simulink library "vehdynlibeom_TUM"  (R2018b)
settings: Solver=VariableStepAuto  StartTime=0.0  StopTime=10.0  RelTol=1e-3
libraries: autolibsharedcommon x7, shared6dof x4, shared6dofsys x3, autolibshared x2, sharedutil x2, sharedtransform x1
Description:
  | Vehicle Dynamics Blockset: Equations of Motion
  | Copyright 2017 The MathWorks Inc.
settings Model: ModifiedByFormat=The MathWorks, Inc.  Creator=The MathWorks, Inc.  LastModifiedBy=The MathWorks, Inc.
settings DebuggingCC: LibraryContextMissingDiagnostic=none
settings SFSimCC: SimUseLocalCustomCode=off
settings RTWCC: RTWUseLocalCustomCode=off
settings CodeAppCC: StateflowObjectComments=on

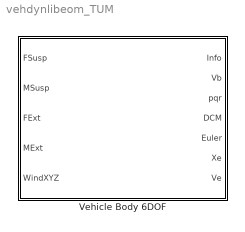
== system vehdynlibeom_TUM ==
  Vehicle Body 6DOF : Subsystem  mask(Vehicle Body 6DOF 2 Axle){m=2000, a=1.4, b=1.6, d=0, h=0.35, Xe0=0, Ye0=0, Ze0=0, vx0_mps=0, vy0_mps=0, vz0_mps=0, phi0_rad=0, theta0_rad=0, psi0_rad=0, phidot0_radps=0, thetadot0_radps=0, psidot0_radps=0, Iveh=[430 0 0; 0 1900 0; 0 0 2100], tw_front=1.8, tw_rear=1.9, z1m=0, z1R=[-.25,.125,.15], z1I=[1.4,-.2,.1;-.2,1.4,.1;.1,.1,2.25].*0, z2m=0, z2R=[1.4,0,.8], z2I=[1.4,-.2,.1;-.2,1.4,.1;.1,.1,2.25].*0, z3m=0, z3R=[.75,-.5,.4], z3I=[5,-.1,-2;-2,9,.1;-.1,.1,6].*0, z4m=0, z4R=[.75,.5,.4], z4I=[5,-.1,-2;-2,9,.1;-.1,.1,6].*0, z5m=0, z5R=[1.25,-.5,.4], z5I=[5,-.1,-2;-2,9,.1;-.1,.1,6].*0, z6m=0, z6R=[1.25,-.5,.4], z6I=[5,-.1,-2;-2,9,.1;-.1,.1,6].*0, z7m=0, z7R=[2,0,.25], z7I=[1.4,-.2,.1;-.2,1.4,.1;.1,.1,2.25].*0, Af=2, Cd=.3, Cl=.1, Cpm=.1, beta_w=[0:0.001:0.01], Cs=[0:0.01:0.1], Cym=[0:0.001:0.01], sign_cl=0, Pabs=101325, Tair=273, g=9.81, xdot_tol=.1, longOff=0, latOff=0, vertOff=0, aMode=2}
      mask prompts: m "vdynblks:vehdynVehBody6Dof:blkPrm_m"; a "vdynblks:vehdynVehBody6Dof:blkPrm_a"; b "vdynblks:vehdynVehBody6Dof:blkPrm_b"; d "vdynblks:vehdynVehBody6Dof:blkPrm_d"; h "vdynblks:vehdynVehBody6Dof:blkPrm_h"; Xe0 "Initial position in intertial frame Xe0_m [m]"; Ye0 "Initial position in intertial frame Ye0_m [m]"; Ze0 "Initial position in intertial frame Ze0_m [m]"; vx0_mps "Initial velocity vx0_mps [m/s]"; vy0_mps "Initial velocity vy0_mps [m/s]"; vz0_mps "Initial velocity vz0_mps [m/s]"; phi0_rad "Initial Euler angle roll, phi0_rad [rad]"; theta0_rad "Initial Euler angle pitch, theta0_rad [rad]"; psi0_rad "Initial Euler angle yaw, psi0_rad [rad]"; phidot0_radps "Initial body rotation rates phidot0_radps [rad/s]"; thetadot0_radps "Initial body rotation rates theta0_radps [rad/s]"; psidot0_radps "Initial body rotation rates psidot0_radps [rad/s]"; Iveh "vdynblks:vehdynVehBody6Dof:blkPrm_Iveh"; tw_front "Track width front, tw_front [m];"; tw_rear "Track width rear, tw_rear [m];"; z1m "vdynblks:vehdynVehBody6Dof:blkPrm_z1m"; z1R "vdynblks:vehdynVehBody6Dof:blkPrm_z1R"; z1I "vdynblks:vehdynVehBody6Dof:blkPrm_z1I"; z2m "vdynblks:vehdynVehBody6Dof:blkPrm_z2m"; z2R "vdynblks:vehdynVehBody6Dof:blkPrm_z2R"; z2I "vdynblks:vehdynVehBody6Dof:blkPrm_z2I"; z3m "vdynblks:vehdynVehBody6Dof:blkPrm_z3m"; z3R "vdynblks:vehdynVehBody6Dof:blkPrm_z3R"; z3I "vdynblks:vehdynVehBody6Dof:blkPrm_z3I"; z4m "vdynblks:vehdynVehBody6Dof:blkPrm_z4m"; z4R "vdynblks:vehdynVehBody6Dof:blkPrm_z4R"; z4I "vdynblks:vehdynVehBody6Dof:blkPrm_z4I"; z5m "vdynblks:vehdynVehBody6Dof:blkPrm_z5m"; z5R "vdynblks:vehdynVehBody6Dof:blkPrm_z5R"; z5I "vdynblks:vehdynVehBody6Dof:blkPrm_z5I"; z6m "vdynblks:vehdynVehBody6Dof:blkPrm_z6m"; z6R "vdynblks:vehdynVehBody6Dof:blkPrm_z6R"; z6I "vdynblks:vehdynVehBody6Dof:blkPrm_z6I"; z7m "vdynblks:vehdynVehBody6Dof:blkPrm_z7m"; z7R "vdynblks:vehdynVehBody6Dof:blkPrm_z7R"; z7I "vdynblks:vehdynVehBody6Dof:blkPrm_z7I"; Af "vdynblks:vehdynVehBody6Dof:blkPrm_Af"; Cd "vdynblks:vehdynVehBody6Dof:blkPrm_Cd"; Cl "vdynblks:vehdynVehBody6Dof:blkPrm_Cl"; Cpm "vdynblks:vehdynVehBody6Dof:blkPrm_Cpm"; beta_w "vdynblks:vehdynVehBody6Dof:blkPrm_beta_w"; Cs "vdynblks:vehdynVehBody6Dof:blkPrm_Cs"; Cym "vdynblks:vehdynVehBody6Dof:blkPrm_Cym"; sign_cl "Long. lift coeff. sign, sign_cl [-]:"; Pabs "vdynblks:vehdynVehBody6Dof:blkPrm_Pabs"; Tair "vdynblks:vehdynVehBody6Dof:blkPrm_Tair"; g "vdynblks:vehdynVehBody6Dof:blkPrm_g"; xdot_tol "vdynblks:vehdynVehBody6Dof:blkPrm_xdot_tol"; longOff "vdynblks:vehdynVehBody6Dof:blkPrm_longOff"; latOff "vdynblks:vehdynVehBody6Dof:blkPrm_latOff"; vertOff "vdynblks:vehdynVehBody6Dof:blkPrm_vertOff"
      mask help: vdynblks:vehdynVehBody6Dof:blkDesc
      mask init:
      | dummy = 1;
      mask Help: eval('vdynblkshelp(''vb6dof'')')
      mask DialogControl vehLayoutPanel Prompt: vdynblks:vehdynVehBody6Dof:blkDlg_Container28
      mask DialogControl LongPanel Prompt: vdynblks:vehdynVehBody6Dof:blkDlg_LongPanel
      mask DialogControl m Prompt: Vehicle mass, m [kg]:
      mask DialogControl a Prompt: Longitudinal distance from center of mass to front axle, a [m]:
      mask DialogControl b Prompt: Longitudinal distance from center of mass to rear axle, b [m]:
      mask DialogControl d Prompt: Lateral distance from geometric centerline to center of mass, d [m]:
      mask DialogControl h Prompt: Vertical distance from center of mass to axle plane, h [m]:
      mask DialogControl Iveh Prompt: Chassis inertia tensor, Iveh [kg*m^2]:
      mask DialogControl loadPanel Prompt: vdynblks:vehdynVehBody6Dof:blkDlg_loadPanel
      mask DialogControl zone1Panel Prompt: vdynblks:vehdynVehBody6Dof:blkDlg_zone1Panel
      mask DialogControl z1m Prompt: Mass, z1m [kg]:
      mask DialogControl z1R Prompt: Distance vector from front axle, z1R [m]:
      mask DialogControl z1I Prompt: Inertia tensor, z1I, [kg*m^2]:
      mask DialogControl zone2Panel Prompt: vdynblks:vehdynVehBody6Dof:blkDlg_zone2Panel
      mask DialogControl z2m Prompt: Mass, z2m [kg]:
      mask DialogControl z2R Prompt: Distance vector from front axle, z2R [m]:
      mask DialogControl z2I Prompt: Inertia tensor, z2I, [kg*m^2]:
      mask DialogControl zone3Panel Prompt: vdynblks:vehdynVehBody6Dof:blkDlg_zone3Panel
      mask DialogControl z3m Prompt: Mass, z3m [kg]:
      mask DialogControl z3R Prompt: Distance vector from front axle, z3R [m]:
      mask DialogControl z3I Prompt: Inertia tensor, z3I, [kg*m^2]:
      mask DialogControl zone4Panel Prompt: vdynblks:vehdynVehBody6Dof:blkDlg_zone4Panel
      mask DialogControl z4m Prompt: Mass, z4m [kg]:
      mask DialogControl z4R Prompt: Distance vector from front axle, z4R [m]:
      mask DialogControl z4I Prompt: Inertia tensor, z4I, [kg*m^2]:
      mask DialogControl zone5Panel Prompt: vdynblks:vehdynVehBody6Dof:blkDlg_zone5Panel
      mask DialogControl z5m Prompt: Mass, z5m [kg]:
      mask DialogControl z5R Prompt: Distance vector from front axle, z5R [m]:
      mask DialogControl z5I Prompt: Inertia tensor, z5I, [kg*m^2]:
      mask DialogControl zone6Panel Prompt: vdynblks:vehdynVehBody6Dof:blkDlg_zone6Panel
      mask DialogControl z6m Prompt: Mass, z6m [kg]:
      mask DialogControl z6R Prompt: Distance vector from front axle, z6R [m]:
      mask DialogControl z6I Prompt: Inertia tensor, z6I, [kg*m^2]:
      mask DialogControl zone7Panel Prompt: vdynblks:vehdynVehBody6Dof:blkDlg_zone7Panel
      mask DialogControl z7m Prompt: Mass, z7m [kg]:
      mask DialogControl z7R Prompt: Distance vector from front axle, z7R [m]:
      mask DialogControl z7I Prompt: Inertia tensor, z7I, [kg*m^2]:
      mask DialogControl AeroParams Prompt: vdynblks:vehdynVehBody6Dof:blkDlg_AeroParams
      mask DialogControl Af Prompt: Longitudinal drag area, Af [m^2]:
      mask DialogControl Cd Prompt: Longitudinal drag coefficient, Cd [-]:
      mask DialogControl Cl Prompt: Longitudinal lift coefficient, Cl [-]:
      mask DialogControl Cpm Prompt: Longitudinal drag pitch moment, Cpm [-]:
      mask DialogControl beta_w Prompt: Relative wind angle vector, beta_w [rad]:
      mask DialogControl Cs Prompt: Side force coefficient vector, Cs [-]:
      mask DialogControl Cym Prompt: Yaw moment coefficient vector, Cym [-]:
      mask DialogControl EnviroPanel Prompt: vdynblks:vehdynVehBody6Dof:blkDlg_EnviroPanel
      mask DialogControl Pabs Prompt: Absolute Pressure, Pabs [Pa]:
      mask DialogControl Tair Prompt: Air temperature, Tair [K]:
      mask DialogControl g Prompt: Gravitational acceleration, g [m/s^2]:
      mask DialogControl SimPanel Prompt: vdynblks:vehdynVehBody6Dof:blkDlg_SimPanel
      mask DialogControl xdot_tol Prompt: Longitudinal velocity tolerance, xdot_tol [m/s]:
      mask DialogControl longOff Prompt: Geometric longitudinal offset from axle plane, longOff [m]:
      mask DialogControl latOff Prompt: Geometric lateral offset from axle plane, latOff [m]:
      mask DialogControl vertOff Prompt: Geometric vertical offset from axle plane, vertOff [m]:
      mask Display:
      | try
      |     IconInfo = vehdynicon('vehdynlib6dofcar',gcb,8);
      | 
      |     image(IconInfo.image, IconInfo.position);
      | 
      |     for i = 1:numel(IconInfo.lconn)
      |         port_label('lconn', i, IconInfo.lconn{i})
      |     end
      | 
      |     for j = 1:numel(IconInfo.rconn)
      |         port_label('rconn', j, IconInfo.rconn{j})
      |     end
      | 
      |     for k = 1:numel(IconInfo.input)
      |         port_label('input', k, IconInfo.input{k})
      |     end
      | 
      |     for m = 1:numel(IconInfo.output)
      |         port_label('output', m, IconInfo.output{m})
      |     end
      | catch
      |     fprintf('Vehicle Body \n 6DOF Car')
      | end

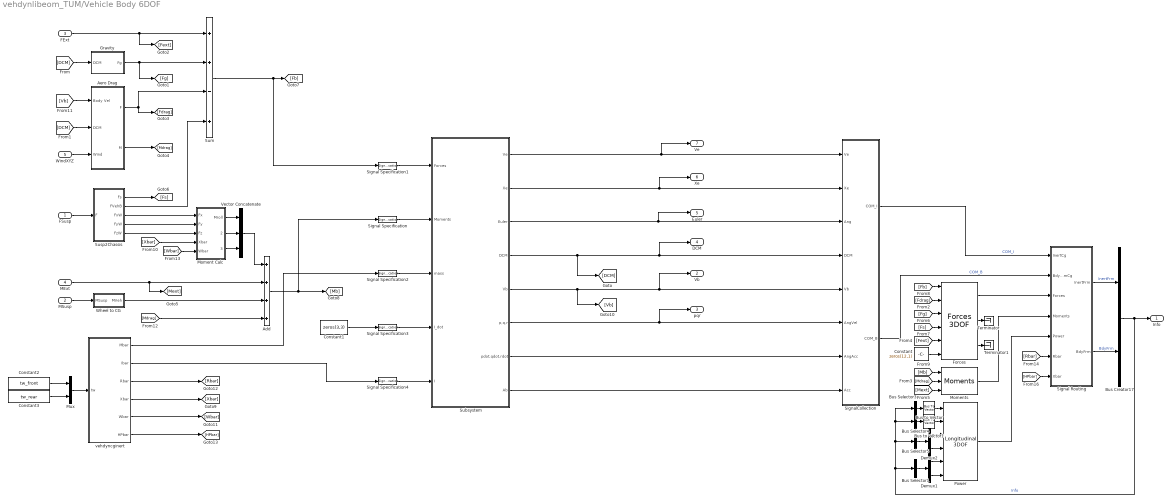
== system vehdynlibeom_TUM/Vehicle Body 6DOF ==
  FSusp : Inport  Unit=N
  MSusp : Inport  Port=2  Unit=N*m
  FExt : Inport  Port=3  Unit=N
  MExt : Inport  Port=4  Unit=N*m
  WindXYZ : Inport  Port=5  Unit=m/s
  Add : Sum  Inputs=++++
  Aero Drag : Subsystem
  Bus Creator17 : BusCreator  Inputs=2
  Bus Selector1 : BusSelector  OutputSignals=BdyFrm.Moments.Body.Mx,BdyFrm.Moments.Body.My,BdyFrm.Moments.Body.Mz,BdyFrm.Cg.AngVel.p,BdyFrm.Cg.AngVel.q,BdyFrm.Cg.AngVel.r  OutputAsBus=on
  Bus Selector3 : BusSelector  OutputSignals=BdyFrm.Forces.Body.Fx,BdyFrm.Forces.Body.Fy,BdyFrm.Forces.Body.Fz  OutputAsBus=on
  Bus Selector4 : BusSelector  OutputSignals=BdyFrm.Forces.Drag.Fx,BdyFrm.Forces.Drag.Fy,BdyFrm.Forces.Drag.Fz  OutputAsBus=on
  Bus Selector5 : BusSelector  OutputSignals=BdyFrm.Cg.Vel.xdot,BdyFrm.Cg.Vel.ydot,BdyFrm.Cg.Vel.zdot,BdyFrm.Moments.Drag.Mx,BdyFrm.Moments.Drag.My,BdyFrm.Moments.Drag.Mz  OutputAsBus=on
  Bus to Vector : BusToVector
  Bus to Vector1 : BusToVector
  Constant : Constant  Value=zeros(12,1)
  Constant1 : Constant  Value=zeros(3,3)
  Constant2 : Constant  Value=tw_front
  Constant3 : Constant  Value=tw_rear
  Demux1 : Demux  Outputs=[3, 3]
  Demux2 : Demux  Outputs=[3, 3]
  Forces : autolibshared/Vehicle Body 3DOF Single Track/Signal Routing/Signal Routing Dual/Forces 3DOF  SystemSampleTime=-1  VariantControl=2
      settings: SourceProductName=Powertrain Blockset  SourceProductBaseCode=PW
  Gravity : Subsystem
  Moment Calc : Subsystem
  Moments : autolibsharedcommon/Bus Creation/Moments  SystemSampleTime=-1
      settings: SourceProductName=Powertrain Blockset  SourceProductBaseCode=PW
  Mux : Mux  Inputs=2
  Power : autolibsharedcommon/Bus Creation/Power/Longitudinal 3DOF  SystemSampleTime=-1  VariantControl=2
      settings: SourceProductName=Powertrain Blockset  SourceProductBaseCode=PW
  Signal Routing : Subsystem  VariantControl=2
  Signal Specification : SignalSpecification  Dimensions=[3,1]
  Signal Specification1 : SignalSpecification  Dimensions=[3,1]
  Signal Specification2 : SignalSpecification  Dimensions=[1,1]
  Signal Specification3 : SignalSpecification  Dimensions=[3,3]
  Signal Specification4 : SignalSpecification  Dimensions=[3,3]
  SignalCollection : Subsystem
  Subsystem : Subsystem
  Sum : Sum  Inputs=++-+  SaturateOnIntegerOverflow=on  InputSameDT=on  OutDataTypeStr=Inherit: Same as first input
  Susp2Chassis : Subsystem
  Terminator : Terminator
  Terminator1 : Terminator
  Vector Concatenate : Concatenate  NumInputs=3
  Wheel to CG : Subsystem
  vehdyncginert : MATLAB Function  TreatAsAtomicUnit=on
  Info : Outport
  Vb : Outport  Port=2  Unit=m/s
  pqr : Outport  Port=3  Unit=rad/s
  DCM : Outport  Port=4
  Euler : Outport  Port=5  Unit=rad
  Xe : Outport  Port=6  Unit=m
  Ve : Outport  Port=7  Unit=m/s
  wires:
  Vector Concatenate/1 -> Add/1
  Susp2Chassis/1(Fs) -> [Fs]
  Moment Calc/3(Myaw) -> Vector Concatenate/3
  Moment Calc/1(Mroll) -> Vector Concatenate/1
  Moment Calc/2(Mpitch) -> Vector Concatenate/2
  MSusp/1 -> Wheel to CG/1(MSusp)
  FSusp/1 -> Susp2Chassis/1(F)
  Gravity/1(Fg) -> Sum/2, [Fg]
  Subsystem/7(pdot,qdot,rdot) -> SignalCollection/7(AngAcc)
  [DCM] -> Gravity/1(DCM)
  WindXYZ/1 -> Aero Drag/3(Wind)
  [Vb] -> Aero Drag/1(Body Vel)
  Add/1 -> [Mb], Signal Specification/1
  Subsystem/4(DCM) -> DCM/1, SignalCollection/4(DCM), [DCM]
  Aero Drag/2(M) -> [Mdrag]
  Aero Drag/1(F) -> [Fdrag], Sum/3
  [DCM] -> Aero Drag/2(DCM)
  Sum/1 -> Signal Specification1/1, [Fb]
  Subsystem/8(Ab) -> SignalCollection/8(Acc)
  FExt/1 -> [Fext], Sum/1
  Bus Selector1/1 -> Demux1/1
  Bus Selector3/1 -> Bus to Vector/1
  Demux2/2 -> Power/4
  Bus to Vector/1 -> Power/1
  Bus Selector5/1 -> Demux2/1
  Bus to Vector1/1 -> Power/2
  Demux2/1 -> Power/3
  Bus Selector4/1 -> Bus to Vector1/1
  Bus Creator17/1 -> Bus Selector3/1, Bus Selector4/1, Bus Selector5/1, Bus Selector1/1, Info/1  "Info"
  Demux1/2 -> Power/6
  Signal Routing/1(InertFrm) -> Bus Creator17/1  "InertFrm"
  Demux1/1 -> Power/5
  Power/1 -> Signal Routing/5(Power)
  Signal Routing/2(BdyFrm) -> Bus Creator17/2  "BdyFrm"
  SignalCollection/1(COM_I) -> Signal Routing/1(InertCg)  "COM_I"
  SignalCollection/2(COM_B) -> Signal Routing/2(BdyFrmCg)  "COM_B"
  Forces/1 -> Signal Routing/3(Forces)
  Moments/1 -> Signal Routing/4(Moments)
  [Fdrag] -> Forces/2
  [Mdrag] -> Moments/2
  [Fext] -> Forces/5
  [Mext] -> Moments/3
  [Fg] -> Forces/3
  [Fb] -> Forces/1
  [Mb] -> Moments/1
  Constant/1 -> Forces/6
  Forces/2 -> Terminator/1
  Forces/3 -> Terminator1/1
  Susp2Chassis/2(FVehB) -> Sum/4
  MExt/1 -> [Mext], Add/2
  Wheel to CG/1(MVeh) -> Add/3
  [Fs] -> Forces/4
  Susp2Chassis/3(FxW) -> Moment Calc/1(Fx)
  Susp2Chassis/4(FyW) -> Moment Calc/2(Fy)
  Susp2Chassis/5(FzW) -> Moment Calc/3(Fz)
  Subsystem/3(Euler) -> Euler/1, SignalCollection/3(Ang)
  Subsystem/5(Vb) -> SignalCollection/5(Vb), Vb/1, [Vb]
  Subsystem/6(p,q,r) -> SignalCollection/6(AngVel), pqr/1
  Subsystem/1(Ve) -> Ve/1, SignalCollection/1(Ve)
  Subsystem/2(Xe) -> Xe/1, SignalCollection/2(Xe)
  [Mdrag] -> Add/4
  vehdyncginert/1(Mbar) -> Signal Specification2/1
  vehdyncginert/3(Rbar) -> [Rbar]
  Constant1/1 -> Signal Specification3/1
  vehdyncginert/2(Ibar) -> Signal Specification4/1
  [Xbar] -> Moment Calc/4(Xbar)
  vehdyncginert/4(Xbar) -> [Xbar]
  vehdyncginert/5(Wbar) -> [Wbar]
  [Wbar] -> Moment Calc/5(Wbar)
  [HPbar] -> Signal Routing/7(Xbar)
  vehdyncginert/6(HPbar) -> [HPbar]
  [Rbar] -> Signal Routing/6(Rbar)
  Constant2/1 -> Mux/1
  Constant3/1 -> Mux/2
  Mux/1 -> vehdyncginert/1(tw)
  Signal Specification/1 -> Subsystem/2(Moments)
  Signal Specification1/1 -> Subsystem/1(Forces)
  Signal Specification2/1 -> Subsystem/3(mass)
  Signal Specification3/1 -> Subsystem/4(I_dot)
  Signal Specification4/1 -> Subsystem/5(I)

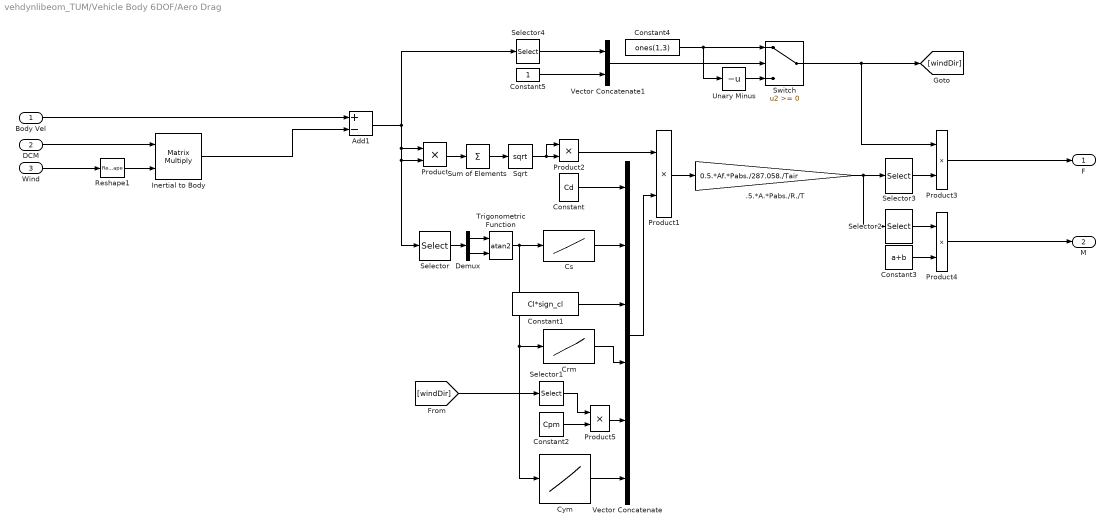
== system vehdynlibeom_TUM/Vehicle Body 6DOF/Aero Drag ==
  Body Vel : Inport
  DCM : Inport  Port=2
  Wind : Inport  Port=3
  .5.*A.*Pabs./R./T : Gain  Gain=0.5.*Af.*Pabs./287.058./Tair
  Add1 : Sum  Inputs=+-
  Constant : Constant  Value=Cd
  Constant1 : Constant  Value=Cl*sign_cl
  Constant2 : Constant  Value=Cpm
  Constant3 : Constant  Value=a+b
  Constant4 : Constant  Value=ones(1,3)
  Constant5 : Constant
  Crm : Lookup_n-D  NumberOfTableDimensions=1  BreakpointsForDimension1=[-1 1]  Table=[0 0]  InternalRulePriority=Speed  RndMeth=Simplest  InputSameDT=on
  Cs : Lookup_n-D  NumberOfTableDimensions=1  BreakpointsForDimension1=beta_w  Table=Cs  ExtrapMethod=Clip  InternalRulePriority=Speed  RndMeth=Simplest  InputSameDT=on
  Cym : Lookup_n-D  NumberOfTableDimensions=1  BreakpointsForDimension1=beta_w  Table=Cym  InternalRulePriority=Speed  RndMeth=Simplest  InputSameDT=on
  Demux : Demux  Outputs=2
  Inertial to Body : Product  Multiplication=Matrix(*)  SaturateOnIntegerOverflow=on  InputSameDT=on  OutDataTypeStr=Inherit: Same as first input
  Product{,1..5} (6 alike) : Product
  Reshape1 : Reshape
  Selector : Selector  InputPortWidth=3  IndexOptions=Index vector (dialog)  Indices=[2 1]  OutputSizes=1
  Selector1 : Selector  InputPortWidth=3  IndexOptions=Index vector (dialog)  Indices=[1]  OutputSizes=1
  Selector2 : Selector  InputPortWidth=6  IndexOptions=Index vector (dialog)  Indices=[4:6]  OutputSizes=1
  Selector3 : Selector  InputPortWidth=6  IndexOptions=Index vector (dialog)  Indices=[1:3]  OutputSizes=1
  Selector4 : Selector  InputPortWidth=3  IndexOptions=Index vector (dialog)  Indices=[1:2]  OutputSizes=1
  Sqrt : Sqrt  SaturateOnIntegerOverflow=on
  Sum of Elements : Sum  Inputs=+
  Switch : Switch  ZeroCross=off
  Trigonometric Function : Trigonometry  Operator=atan2  OutputSignalType=real
  Unary Minus : UnaryMinus
  Vector Concatenate : Concatenate  NumInputs=6
  Vector Concatenate1 : Concatenate
  F : Outport
  M : Outport  Port=2
  wires:
  Reshape1/1 -> Inertial to Body/2
  DCM/1 -> Inertial to Body/1
  Wind/1 -> Reshape1/1
  Constant4/1 -> Switch/1, Unary Minus/1
  Vector Concatenate1/1 -> Switch/2
  Crm/1 -> Vector Concatenate/4
  Constant5/1 -> Vector Concatenate1/2
  Selector3/1 -> Product3/2
  Unary Minus/1 -> Switch/3
  Add1/1 -> Selector4/1, Product/1, Product/2, Selector/1
  Product5/1 -> Vector Concatenate/5
  Vector Concatenate/1 -> Product1/2
  Selector4/1 -> Vector Concatenate1/1
  Demux/2 -> Trigonometric Function/2
  Trigonometric Function/1 -> Cym/1, Crm/1, Cs/1
  Switch/1 -> Product3/1, [windDir]
  Constant1/1 -> Vector Concatenate/3
  Product1/1 -> .5.*A.*Pabs./R./T/1
  Selector2/1 -> Product4/1
  Cs/1 -> Vector Concatenate/2
  Constant/1 -> Vector Concatenate/1
  Product/1 -> Sum of Elements/1
  Selector/1 -> Demux/1
  [windDir] -> Selector1/1
  Sum of Elements/1 -> Sqrt/1
  Constant2/1 -> Product5/2
  Product2/1 -> Product1/1
  Selector1/1 -> Product5/1
  .5.*A.*Pabs./R./T/1 -> Selector2/1, Selector3/1
  Constant3/1 -> Product4/2
  Cym/1 -> Vector Concatenate/6
  Product3/1 -> F/1
  Body Vel/1 -> Add1/1
  Inertial to Body/1 -> Add1/2
  Demux/1 -> Trigonometric Function/1
  Product4/1 -> M/1
  Sqrt/1 -> Product2/2, Product2/1

== system vehdynlibeom_TUM/Vehicle Body 6DOF/Gravity ==
  DCM : Inport
  Inertial gravity vector : Constant  Value=[0; 0; 9.81]
  Inertial to Body : Product  Multiplication=Matrix(*)  SaturateOnIntegerOverflow=on  InputSameDT=on  OutDataTypeStr=Inherit: Same as first input
  Reshape : Reshape
  mass : Gain  Gain=m  SaturateOnIntegerOverflow=on  OutDataTypeStr=Inherit: Same as input  ParamDataTypeStr=Inherit: Same as input
  Fg : Outport
  wires:
  DCM/1 -> Inertial to Body/1
  mass/1 -> Reshape/1  "Fg_I"
  Reshape/1 -> Inertial to Body/2
  Inertial gravity vector/1 -> mass/1
  Inertial to Body/1 -> Fg/1  "Fg_B"

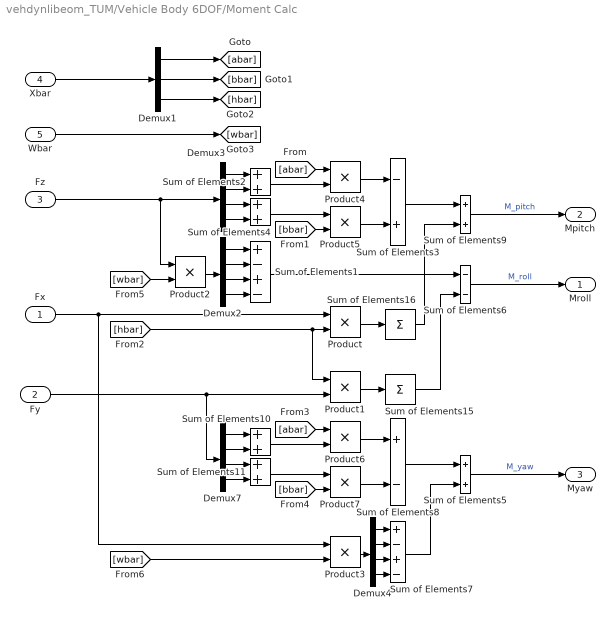
== system vehdynlibeom_TUM/Vehicle Body 6DOF/Moment Calc ==
  Fx : Inport
  Fy : Inport  Port=2
  Fz : Inport  Port=3
  Xbar : Inport  Port=4
  Wbar : Inport  Port=5
  Demux1 : Demux  Outputs=3
  Demux{2..4,7} (4 alike) : Demux
  Product{,1..7} (8 alike) : Product
  Sum of Elements1 : Sum  Inputs=+-+-
  Sum of Elements{2,4..5,9..11} (6 alike) : Sum
  Sum of Elements15 : Sum  Inputs=+
  Sum of Elements16 : Sum  Inputs=+
  Sum of Elements3 : Sum  Inputs=-+
  Sum of Elements6 : Sum  Inputs=--
  Sum of Elements7 : Sum  Inputs=+-+-
  Sum of Elements8 : Sum  Inputs=+-
  Mroll : Outport
  Mpitch : Outport  Port=2
  Myaw : Outport  Port=3
  wires:
  Product1/1 -> Sum of Elements15/1
  Product/1 -> Sum of Elements16/1
  Sum of Elements6/1 -> Mroll/1  "M_roll"
  Sum of Elements9/1 -> Mpitch/1  "M_pitch"
  Product4/1 -> Sum of Elements3/1
  Demux2/1 -> Sum of Elements1/1
  Sum of Elements7/1 -> Sum of Elements5/2
  Product5/1 -> Sum of Elements3/2
  Sum of Elements16/1 -> Sum of Elements9/2
  Sum of Elements5/1 -> Myaw/1  "M_yaw"
  Sum of Elements8/1 -> Sum of Elements5/1
  Sum of Elements15/1 -> Sum of Elements6/2
  Demux3/2 -> Sum of Elements2/2
  Demux3/1 -> Sum of Elements2/1
  Demux3/4 -> Sum of Elements4/2
  [hbar] -> Product1/1, Product/2
  Sum of Elements3/1 -> Sum of Elements9/1
  Demux3/3 -> Sum of Elements4/1
  Sum of Elements4/1 -> Product5/1
  Sum of Elements2/1 -> Product4/2
  Sum of Elements1/1 -> Sum of Elements6/1
  Fz/1 -> Product2/1, Demux3/1
  Fx/1 -> Product3/1, Product/1
  Demux2/4 -> Sum of Elements1/4
  Demux4/4 -> Sum of Elements7/4
  Demux4/1 -> Sum of Elements7/1
  Fy/1 -> Demux7/1, Product1/2
  Demux2/2 -> Sum of Elements1/2
  Demux2/3 -> Sum of Elements1/3
  Product2/1 -> Demux2/1
  Demux4/2 -> Sum of Elements7/2
  Demux4/3 -> Sum of Elements7/3
  Product3/1 -> Demux4/1
  [wbar] -> Product3/2
  [abar] -> Product4/1
  [bbar] -> Product5/2
  [bbar] -> Product7/2
  [abar] -> Product6/1
  Sum of Elements10/1 -> Product6/2
  Sum of Elements11/1 -> Product7/1
  Product7/1 -> Sum of Elements8/2
  Product6/1 -> Sum of Elements8/1
  Demux7/3 -> Sum of Elements11/1
  Demux7/4 -> Sum of Elements11/2
  Demux7/1 -> Sum of Elements10/1
  Demux7/2 -> Sum of Elements10/2
  Demux1/3 -> [hbar]
  Xbar/1 -> Demux1/1
  [wbar] -> Product2/2
  Demux1/2 -> [bbar]
  Demux1/1 -> [abar]
  Wbar/1 -> [wbar]

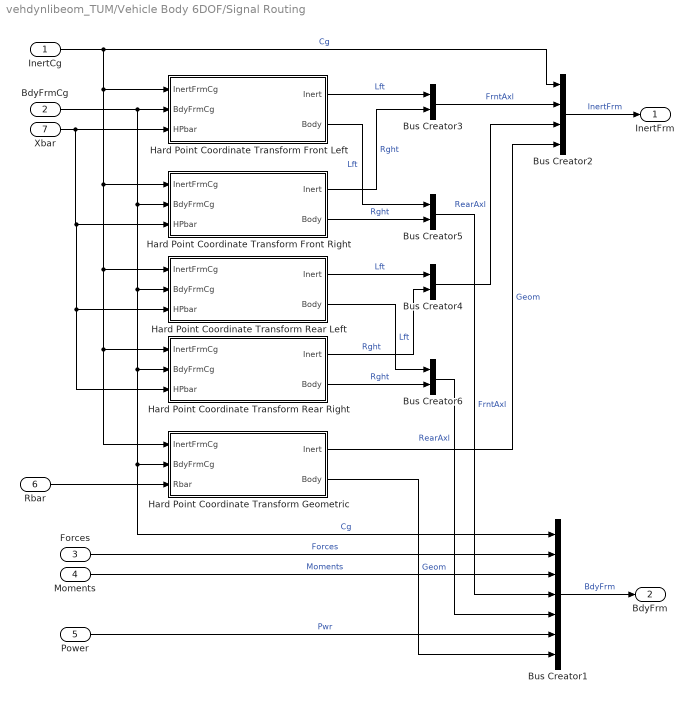
== system vehdynlibeom_TUM/Vehicle Body 6DOF/Signal Routing ==
  InertCg : Inport
  BdyFrmCg : Inport  Port=2
  Forces : Inport  Port=3
  Moments : Inport  Port=4
  Power : Inport  Port=5
  Rbar : Inport  Port=6
  Xbar : Inport  Port=7
  Bus Creator1 : BusCreator  Inputs=7
  Bus Creator2 : BusCreator  Inputs=4
  Bus Creator{3..6} (4 alike) : BusCreator  Inputs=2
  Hard Point Coordinate Transform Front Left : Subsystem
  Hard Point Coordinate Transform Front Right : Subsystem
  Hard Point Coordinate Transform Geometric : Subsystem
  Hard Point Coordinate Transform Rear Left : Subsystem
  Hard Point Coordinate Transform Rear Right : Subsystem
  InertFrm : Outport
  BdyFrm : Outport  Port=2
  wires:
  Hard Point Coordinate Transform Geometric/1(Inert) -> Bus Creator2/4  "Geom"
  Hard Point Coordinate Transform Geometric/2(Body) -> Bus Creator1/7  "Geom"
  Power/1 -> Bus Creator1/6  "Pwr"
  Forces/1 -> Bus Creator1/2  "Forces"
  BdyFrmCg/1 -> Hard Point Coordinate Transform Geometric/2(BdyFrmCg), Bus Creator1/1, Hard Point Coordinate Transform Rear Right/2(BdyFrmCg), Hard Point Coordinate Transform Rear Left/2(BdyFrmCg), Hard Point Coordinate Transform Front Right/2(BdyFrmCg), Hard Point Coordinate Transform Front Left/2(BdyFrmCg)  "Cg"
  Bus Creator3/1 -> Bus Creator2/2  "FrntAxl"
  Bus Creator1/1 -> BdyFrm/1  "BdyFrm"
  Bus Creator2/1 -> InertFrm/1  "InertFrm"
  Bus Creator4/1 -> Bus Creator2/3  "RearAxl"
  InertCg/1 -> Hard Point Coordinate Transform Rear Left/1(InertFrmCg), Hard Point Coordinate Transform Rear Right/1(InertFrmCg), Hard Point Coordinate Transform Geometric/1(InertFrmCg), Hard Point Coordinate Transform Front Right/1(InertFrmCg), Hard Point Coordinate Transform Front Left/1(InertFrmCg), Bus Creator2/1  "Cg"
  Bus Creator5/1 -> Bus Creator1/4  "FrntAxl"
  Moments/1 -> Bus Creator1/3  "Moments"
  Hard Point Coordinate Transform Front Left/1(Inert) -> Bus Creator3/1  "Lft"
  Hard Point Coordinate Transform Front Right/1(Inert) -> Bus Creator3/2  "Rght"
  Hard Point Coordinate Transform Rear Left/1(Inert) -> Bus Creator4/1  "Lft"
  Hard Point Coordinate Transform Rear Right/1(Inert) -> Bus Creator4/2  "Rght"
  Hard Point Coordinate Transform Rear Right/2(Body) -> Bus Creator6/2  "Rght"
  Hard Point Coordinate Transform Rear Left/2(Body) -> Bus Creator6/1  "Lft"
  Hard Point Coordinate Transform Front Right/2(Body) -> Bus Creator5/2  "Rght"
  Hard Point Coordinate Transform Front Left/2(Body) -> Bus Creator5/1  "Lft"
  Bus Creator6/1 -> Bus Creator1/5  "RearAxl"
  Xbar/1 -> Hard Point Coordinate Transform Front Right/3(HPbar), Hard Point Coordinate Transform Rear Right/3(HPbar), Hard Point Coordinate Transform Rear Left/3(HPbar), Hard Point Coordinate Transform Front Left/3(HPbar)
  Rbar/1 -> Hard Point Coordinate Transform Geometric/3(Rbar)

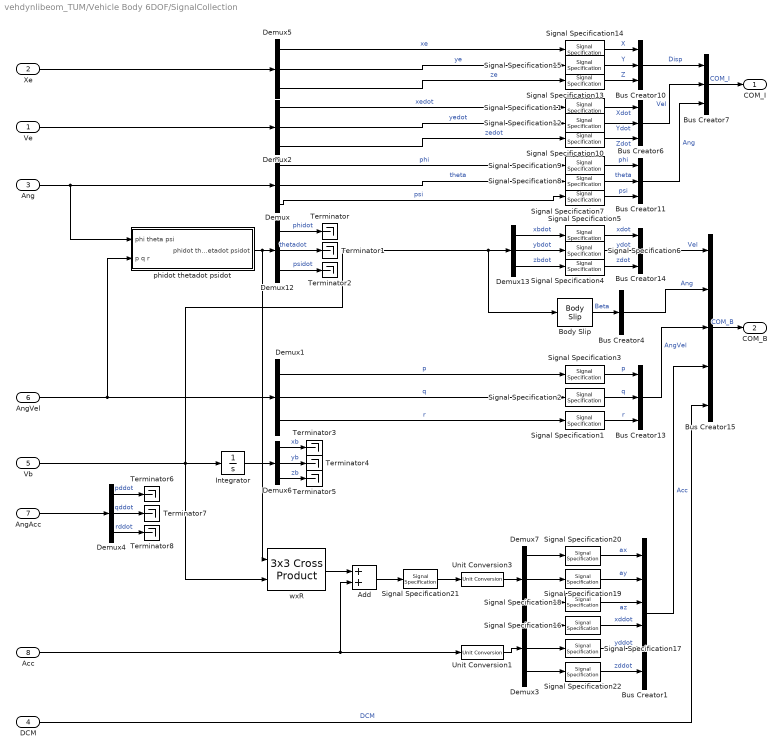
== system vehdynlibeom_TUM/Vehicle Body 6DOF/SignalCollection ==
  Ve : Inport
  Xe : Inport  Port=2
  Ang : Inport  Port=3
  DCM : Inport  Port=4
  Vb : Inport  Port=5
  AngVel : Inport  Port=6
  AngAcc : Inport  Port=7
  Acc : Inport  Port=8
  Add : Sum
  Body Slip : autolibshared/Vehicle Body 3DOF Single Track/Signal Routing/Signal Routing/state2bus/Body Slip  mask{xdot_tol=xdot_tol}
      mask prompts: xdot_tol "Longituindal low speed tolerance, xdot_tol [m/s]:"
      settings: SourceProductName=Powertrain Blockset  SourceProductBaseCode=PW
  Bus Creator1 : BusCreator  Inputs=6
  Bus Creator{6..7,10..11,13..14} (6 alike) : BusCreator  Inputs=3
  Bus Creator15 : BusCreator  Inputs=5
  Bus Creator4 : BusCreator  Inputs=1
  Demux{,1..7,12..13} (10 alike) : Demux  Outputs=3
  Integrator : Integrator
  Signal Specification1 : SignalSpecification  Unit=rad/s
  Signal Specification{4..6,10..12} (6 alike) : SignalSpecification  Unit=m/s
  Signal Specification13 : SignalSpecification  Unit=m
  Signal Specification14 : SignalSpecification  Unit=m
  Signal Specification15 : SignalSpecification  Unit=m
  Signal Specification{16..17,21..22} (4 alike) : SignalSpecification  Unit=m/s^2
  Signal Specification18 : SignalSpecification  Unit=gn
  Signal Specification19 : SignalSpecification  Unit=gn
  Signal Specification2 : SignalSpecification  Unit=rad/s
  Signal Specification20 : SignalSpecification  Unit=gn
  Signal Specification3 : SignalSpecification  Unit=rad/s
  Signal Specification7 : SignalSpecification  Unit=rad
  Signal Specification8 : SignalSpecification  Unit=rad
  Signal Specification9 : SignalSpecification  Unit=rad
  Terminator{,1..8} (9 alike) : Terminator
  Unit Conversion1 : UnitConversion
  Unit Conversion3 : UnitConversion
  phidot thetadot psidot : Subsystem
  wxR : sharedutil/3x3 Cross Product  aMode=aMode
      settings: SourceProductBaseCode=AE
  COM_I : Outport
  COM_B : Outport  Port=2
  wires:
  AngAcc/1 -> Demux4/1
  Demux/1 -> Signal Specification9/1  "phi"
  Demux/2 -> Signal Specification8/1  "theta"
  Demux/3 -> Signal Specification7/1  "psi"
  Demux1/2 -> Signal Specification2/1  "q"
  Demux1/3 -> Signal Specification1/1  "r"
  Demux2/1 -> Signal Specification11/1  "xedot"
  Demux2/2 -> Signal Specification12/1  "yedot"
  Demux2/3 -> Signal Specification10/1  "zedot"
  Demux3/1 -> Signal Specification16/1
  Demux3/2 -> Signal Specification17/1
  Demux3/3 -> Signal Specification22/1
  Xe/1 -> Demux5/1
  Demux5/1 -> Signal Specification14/1  "xe"
  Demux5/2 -> Signal Specification15/1  "ye"
  Demux5/3 -> Signal Specification13/1  "ze"
  Demux4/1 -> Terminator6/1  "pddot"
  Demux4/2 -> Terminator7/1  "qddot"
  Demux4/3 -> Terminator8/1  "rddot"
  Ve/1 -> Demux2/1
  Ang/1 -> Demux/1, phidot thetadot psidot/1(phi theta psi)
  Demux12/1 -> Terminator/1  "phidot"
  Demux12/2 -> Terminator1/1  "thetadot"
  Demux12/3 -> Terminator2/1  "psidot"
  phidot thetadot psidot/1(phidot thetadot psidot) -> wxR/1, Demux12/1
  AngVel/1 -> phidot thetadot psidot/2(p q r), Demux1/1
  Demux13/1 -> Signal Specification5/1  "xbdot"
  Demux13/2 -> Signal Specification6/1  "ybdot"
  Demux13/3 -> Signal Specification4/1  "zbdot"
  Vb/1 -> wxR/2, Body Slip/1, Demux13/1, Integrator/1
  Bus Creator7/1 -> COM_I/1  "COM_I"
  Demux1/1 -> Signal Specification3/1  "p"
  Integrator/1 -> Demux6/1
  Demux6/1 -> Terminator3/1  "xb"
  Demux6/2 -> Terminator4/1  "yb"
  Demux6/3 -> Terminator5/1  "zb"
  Signal Specification9/1 -> Bus Creator11/1  "phi"
  Bus Creator13/1 -> Bus Creator15/3  "AngVel"
  Signal Specification3/1 -> Bus Creator13/1  "p"
  Signal Specification1/1 -> Bus Creator13/3  "r"
  Signal Specification6/1 -> Bus Creator14/2  "ydot"
  Signal Specification7/1 -> Bus Creator11/3  "psi"
  Bus Creator11/1 -> Bus Creator7/3  "Ang"
  Signal Specification4/1 -> Bus Creator14/3  "zdot"
  Bus Creator6/1 -> Bus Creator7/2  "Vel"
  Signal Specification8/1 -> Bus Creator11/2  "theta"
  Bus Creator15/1 -> COM_B/1  "COM_B"
  Signal Specification11/1 -> Bus Creator6/1  "Xdot"
  Signal Specification5/1 -> Bus Creator14/1  "xdot"
  Signal Specification13/1 -> Bus Creator10/3  "Z"
  Signal Specification2/1 -> Bus Creator13/2  "q"
  Signal Specification12/1 -> Bus Creator6/2  "Ydot"
  Signal Specification10/1 -> Bus Creator6/3  "Zdot"
  Bus Creator14/1 -> Bus Creator15/1  "Vel"
  Signal Specification15/1 -> Bus Creator10/2  "Y"
  Signal Specification14/1 -> Bus Creator10/1  "X"
  Bus Creator10/1 -> Bus Creator7/1  "Disp"
  Bus Creator1/1 -> Bus Creator15/4  "Acc"
  Signal Specification18/1 -> Bus Creator1/3  "az"
  Signal Specification20/1 -> Bus Creator1/1  "ax"
  Signal Specification19/1 -> Bus Creator1/2  "ay"
  wxR/1 -> Add/1
  Demux7/2 -> Signal Specification19/1
  Demux7/1 -> Signal Specification20/1
  Demux7/3 -> Signal Specification18/1
  Acc/1 -> Add/2, Unit Conversion1/1
  Add/1 -> Signal Specification21/1
  Unit Conversion3/1 -> Demux7/1
  Signal Specification21/1 -> Unit Conversion3/1
  Unit Conversion1/1 -> Demux3/1
  Signal Specification17/1 -> Bus Creator1/5  "yddot"
  Signal Specification22/1 -> Bus Creator1/6  "zddot"
  Signal Specification16/1 -> Bus Creator1/4  "xddot"
  DCM/1 -> Bus Creator15/5  "DCM"
  Bus Creator4/1 -> Bus Creator15/2  "Ang"
  Body Slip/1 -> Bus Creator4/1  "Beta"

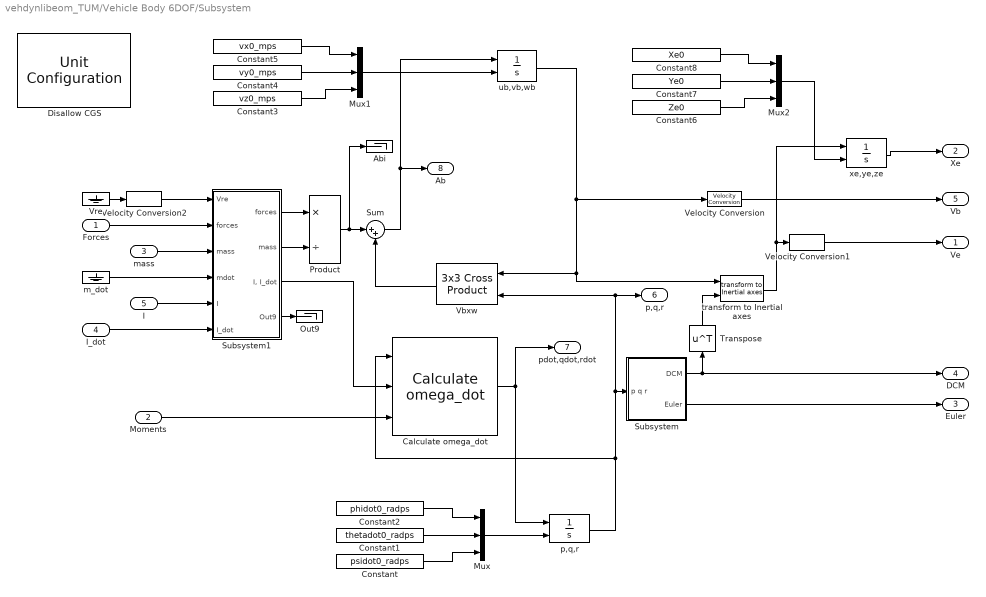
== system vehdynlibeom_TUM/Vehicle Body 6DOF/Subsystem ==
  Forces : Inport  Unit=N  PortDimensions=3
  Moments : Inport  Port=2  Unit=N*m  PortDimensions=3
  mass : Inport  Port=3  Unit=kg  PortDimensions=1
  I_dot : Inport  Port=4  Unit=N*m  PortDimensions=[3,3]
  I : Inport  Port=5  Unit=kg*m^2  PortDimensions=[3,3]
  Abi : Terminator
  Calculate omega_dot : shared6dofsys/Calculate omega_dot  aMode=aMode
      settings: SourceProductName=Aerospace Blockset  SourceProductBaseCode=AE
  Constant : Constant  Value=psidot0_radps
  Constant1 : Constant  Value=thetadot0_radps
  Constant2 : Constant  Value=phidot0_radps
  Constant3 : Constant  Value=vz0_mps
  Constant4 : Constant  Value=vy0_mps
  Constant5 : Constant  Value=vx0_mps
  Constant6 : Constant  Value=Ze0
  Constant7 : Constant  Value=Ye0
  Constant8 : Constant  Value=Xe0
  Disallow CGS : UnitConfiguration  UnitSystemsStr=English,SI,SI (extended)  AllowAllUnitSystems=off
  Mux : Mux  Inputs=3
  Mux1 : Mux  Inputs=3
  Mux2 : Mux  Inputs=3
  Out9 : Terminator
  Product : Product  Inputs=*/  SaturateOnIntegerOverflow=on  OutDataTypeStr=Inherit: Same as first input
  Subsystem : Subsystem
  Subsystem1 : Subsystem
  Sum : Sum  Inputs=|++  SaturateOnIntegerOverflow=on
  Transpose : Math  Operator=transpose  SaturateOnIntegerOverflow=on
  Vbxw : sharedutil/3x3 Cross Product  aMode=aMode
      settings: SourceProductBaseCode=AE
  Velocity Conversion : shared6dof/6DOF (Euler Angles)/Velocity Conversion  SystemSampleTime=-1
      settings: SourceProductName=Aerospace Blockset  SourceProductBaseCode=AE
  Velocity Conversion1 : shared6dof/6DOF (Euler Angles)/Velocity Conversion1  SystemSampleTime=-1
      settings: SourceProductName=Aerospace Blockset  SourceProductBaseCode=AE
  Velocity Conversion2 : shared6dof/6DOF (Euler Angles)/Velocity Conversion2  SystemSampleTime=-1
      settings: SourceProductName=Aerospace Blockset  SourceProductBaseCode=AE
  Vre : Ground
  m_dot : Ground
  "p,q,r " : Integrator  InitialConditionSource=external  InitialCondition=[0,0,0]
  "transform to Inertial axes " : shared6dof/6DOF (Euler Angles)/transform to Inertial axes   SystemSampleTime=-1
      settings: SourceProductName=Aerospace Blockset  SourceProductBaseCode=AE
  ub,vb,wb : Integrator  InitialConditionSource=external  InitialCondition=[0,0,0]
  xe,ye,ze : Integrator  InitialConditionSource=external  InitialCondition=[0,0,0]
  Ve : Outport  Unit=m/s
  Xe : Outport  Port=2  Unit=m
  Euler : Outport  Port=3  Unit=rad
  DCM : Outport  Port=4  Unit=1
  Vb : Outport  Port=5  Unit=m/s
  p,q,r : Outport  Port=6  Unit=rad/s
  pdot,qdot,rdot : Outport  Port=7  Unit=rad/s^2
  Ab : Outport  Port=8  Unit=m/s^2
  wires:
  I/1 -> Subsystem1/5(I)
  Forces/1 -> Subsystem1/2(forces)
  "p,q,r "/1 -> Vbxw/2, p,q,r/1, Subsystem/1("p q r "), Calculate omega_dot/1
  Vre/1 -> Velocity Conversion2/1
  "transform to Inertial axes "/1 -> Velocity Conversion1/1, xe,ye,ze/1
  I_dot/1 -> Subsystem1/6(I_dot)
  Subsystem1/1("forces ") -> Product/1
  Moments/1 -> Calculate omega_dot/3
  Sum/1 -> ub,vb,wb/1, Ab/1
  Velocity Conversion1/1 -> Ve/1
  mass/1 -> Subsystem1/3("mass ")
  Subsystem1/2(mass) -> Product/2
  Calculate omega_dot/1 -> pdot,qdot,rdot/1, "p,q,r "/1
  m_dot/1 -> Subsystem1/4(mdot)
  Velocity Conversion/1 -> Vb/1
  Transpose/1 -> "transform to Inertial axes "/2
  Subsystem/1(DCM) -> DCM/1, Transpose/1
  Vbxw/1 -> Sum/2
  Subsystem/2(Euler) -> Euler/1
  Product/1 -> Abi/1, Sum/1
  xe,ye,ze/1 -> Xe/1
  Velocity Conversion2/1 -> Subsystem1/1(Vre)
  ub,vb,wb/1 -> Vbxw/1, "transform to Inertial axes "/1, Velocity Conversion/1
  Subsystem1/4(Out9) -> Out9/1
  Constant2/1 -> Mux/1
  Constant1/1 -> Mux/2
  Mux/1 -> "p,q,r "/2
  Constant3/1 -> Mux1/3
  Constant5/1 -> Mux1/1
  Constant4/1 -> Mux1/2
  Mux1/1 -> ub,vb,wb/2
  Constant6/1 -> Mux2/3
  Constant8/1 -> Mux2/1
  Constant7/1 -> Mux2/2
  Mux2/1 -> xe,ye,ze/2
  Subsystem1/3("I, I_dot ") -> Calculate omega_dot/2
  Constant/1 -> Mux/3

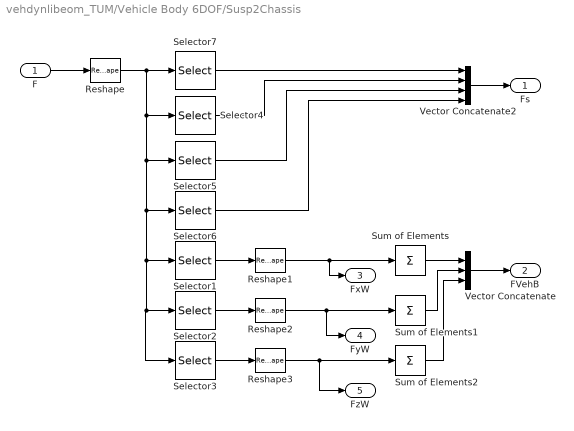
== system vehdynlibeom_TUM/Vehicle Body 6DOF/Susp2Chassis ==
  F : Inport
  Reshape : Reshape  OutputDimensionality=Customize  OutputDimensions=[3,4]
  Reshape1 : Reshape
  Reshape2 : Reshape
  Reshape3 : Reshape
  Selector1 : Selector  NumberOfDimensions=2  InputPortWidth=3  IndexOptions=Index vector (dialog),Select all  Indices=[1],1  OutputSizes=1,1
  Selector2 : Selector  NumberOfDimensions=2  InputPortWidth=3  IndexOptions=Index vector (dialog),Select all  Indices=[2],1  OutputSizes=1,1
  Selector3 : Selector  NumberOfDimensions=2  InputPortWidth=3  IndexOptions=Index vector (dialog),Select all  Indices=[3],1  OutputSizes=1,1
  Selector4 : Selector  NumberOfDimensions=2  InputPortWidth=3  IndexOptions=Select all,Index vector (dialog)  Indices=[1],2  OutputSizes=1,1
  Selector5 : Selector  NumberOfDimensions=2  InputPortWidth=3  IndexOptions=Select all,Index vector (dialog)  Indices=[1],3  OutputSizes=1,1
  Selector6 : Selector  NumberOfDimensions=2  InputPortWidth=3  IndexOptions=Select all,Index vector (dialog)  Indices=[1],4  OutputSizes=1,1
  Selector7 : Selector  NumberOfDimensions=2  InputPortWidth=3  IndexOptions=Select all,Index vector (dialog)  Indices=[1],1  OutputSizes=1,1
  Sum of Elements : Sum  Inputs=+
  Sum of Elements1 : Sum  Inputs=+
  Sum of Elements2 : Sum  Inputs=+
  Vector Concatenate : Concatenate  NumInputs=3
  Vector Concatenate2 : Concatenate  NumInputs=4
  Fs : Outport
  FVehB : Outport  Port=2
  FxW : Outport  Port=3
  FyW : Outport  Port=4
  FzW : Outport  Port=5
  wires:
  F/1 -> Reshape/1
  Sum of Elements/1 -> Vector Concatenate/1
  Sum of Elements1/1 -> Vector Concatenate/2
  Sum of Elements2/1 -> Vector Concatenate/3
  Vector Concatenate/1 -> FVehB/1
  Selector1/1 -> Reshape1/1
  Selector2/1 -> Reshape2/1
  Selector3/1 -> Reshape3/1
  Vector Concatenate2/1 -> Fs/1
  Selector4/1 -> Vector Concatenate2/2
  Selector7/1 -> Vector Concatenate2/1
  Selector5/1 -> Vector Concatenate2/3
  Reshape/1 -> Selector3/1, Selector2/1, Selector1/1, Selector6/1, Selector5/1, Selector4/1, Selector7/1
  Selector6/1 -> Vector Concatenate2/4
  Reshape1/1 -> FxW/1, Sum of Elements/1
  Reshape2/1 -> FyW/1, Sum of Elements1/1
  Reshape3/1 -> FzW/1, Sum of Elements2/1

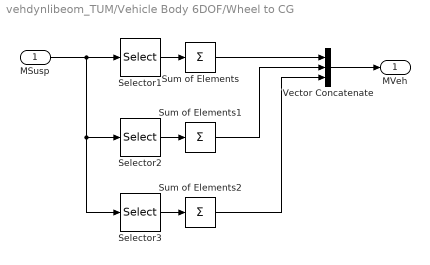
== system vehdynlibeom_TUM/Vehicle Body 6DOF/Wheel to CG ==
  MSusp : Inport
  Selector1 : Selector  NumberOfDimensions=2  InputPortWidth=3  IndexOptions=Index vector (dialog),Select all  Indices=[1],1  OutputSizes=1,1
  Selector2 : Selector  NumberOfDimensions=2  InputPortWidth=3  IndexOptions=Index vector (dialog),Select all  Indices=[2],1  OutputSizes=1,1
  Selector3 : Selector  NumberOfDimensions=2  InputPortWidth=3  IndexOptions=Index vector (dialog),Select all  Indices=[3],1  OutputSizes=1,1
  Sum of Elements : Sum  Inputs=+
  Sum of Elements1 : Sum  Inputs=+
  Sum of Elements2 : Sum  Inputs=+
  Vector Concatenate : Concatenate  NumInputs=3
  MVeh : Outport
  wires:
  Sum of Elements/1 -> Vector Concatenate/1
  Sum of Elements1/1 -> Vector Concatenate/2
  Sum of Elements2/1 -> Vector Concatenate/3
  Vector Concatenate/1 -> MVeh/1
  MSusp/1 -> Selector3/1, Selector2/1, Selector1/1
  Selector2/1 -> Sum of Elements1/1
  Selector1/1 -> Sum of Elements/1
  Selector3/1 -> Sum of Elements2/1

== system vehdynlibeom_TUM/Vehicle Body 6DOF/Signal Routing/Hard Point Coordinate Transform Front Left ==
  InertFrmCg : Inport
  BdyFrmCg : Inport  Port=2
  HPbar : Inport  Port=3
  Hard Point Coordinate Transform External Displacement : autolibsharedcommon/Hard Point Coordinate Transform External Displacement  aMode=aMode
      settings: SourceProductName=Powertrain Blockset  SourceProductBaseCode=PW
  Selector1 : Selector  NumberOfDimensions=2  InputPortWidth=3  IndexOptions=Select all,Index vector (dialog)  Indices=[1],[1]  OutputSizes=1,1
  Inert : Outport
  Body : Outport  Port=2
  wires:
  InertFrmCg/1 -> Hard Point Coordinate Transform External Displacement/1
  Hard Point Coordinate Transform External Displacement/2 -> Body/1
  Selector1/1 -> Hard Point Coordinate Transform External Displacement/3
  BdyFrmCg/1 -> Hard Point Coordinate Transform External Displacement/2
  Hard Point Coordinate Transform External Displacement/1 -> Inert/1
  HPbar/1 -> Selector1/1

== system vehdynlibeom_TUM/Vehicle Body 6DOF/Signal Routing/Hard Point Coordinate Transform Front Right ==
  InertFrmCg : Inport
  BdyFrmCg : Inport  Port=2
  HPbar : Inport  Port=3
  Hard Point Coordinate Transform External Displacement : autolibsharedcommon/Hard Point Coordinate Transform External Displacement  aMode=aMode
      settings: SourceProductName=Powertrain Blockset  SourceProductBaseCode=PW
  Selector1 : Selector  NumberOfDimensions=2  InputPortWidth=3  IndexOptions=Select all,Index vector (dialog)  Indices=[1],[2]  OutputSizes=1,1
  Inert : Outport
  Body : Outport  Port=2
  wires:
  Hard Point Coordinate Transform External Displacement/1 -> Inert/1
  BdyFrmCg/1 -> Hard Point Coordinate Transform External Displacement/2
  Hard Point Coordinate Transform External Displacement/2 -> Body/1
  InertFrmCg/1 -> Hard Point Coordinate Transform External Displacement/1
  HPbar/1 -> Selector1/1
  Selector1/1 -> Hard Point Coordinate Transform External Displacement/3

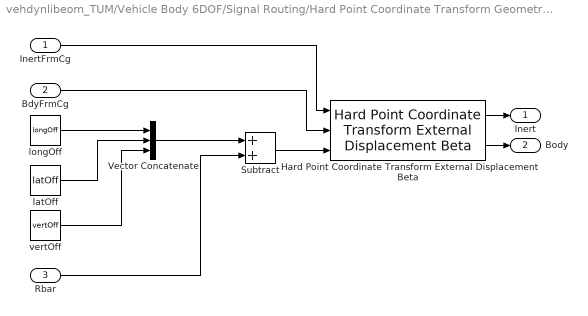
== system vehdynlibeom_TUM/Vehicle Body 6DOF/Signal Routing/Hard Point Coordinate Transform Geometric ==
  InertFrmCg : Inport
  BdyFrmCg : Inport  Port=2
  Rbar : Inport  Port=3
  Hard Point Coordinate Transform External Displacement Beta : autolibsharedcommon/Hard Point Coordinate Transform External Displacement Beta  xdot_tol=xdot_tol  aMode=aMode
      settings: SourceProductName=Powertrain Blockset  SourceProductBaseCode=PW
  Subtract : Sum
  Vector Concatenate : Concatenate  NumInputs=3
  latOff : Constant  Value=latOff
  longOff : Constant  Value=longOff
  "vertOff " : Constant  Value=vertOff
  Inert : Outport
  Body : Outport  Port=2
  wires:
  InertFrmCg/1 -> Hard Point Coordinate Transform External Displacement Beta/1
  Hard Point Coordinate Transform External Displacement Beta/2 -> Body/1
  Vector Concatenate/1 -> Subtract/1
  BdyFrmCg/1 -> Hard Point Coordinate Transform External Displacement Beta/2
  Hard Point Coordinate Transform External Displacement Beta/1 -> Inert/1
  "vertOff "/1 -> Vector Concatenate/3
  longOff/1 -> Vector Concatenate/1
  latOff/1 -> Vector Concatenate/2
  Rbar/1 -> Subtract/2
  Subtract/1 -> Hard Point Coordinate Transform External Displacement Beta/3

== system vehdynlibeom_TUM/Vehicle Body 6DOF/Signal Routing/Hard Point Coordinate Transform Rear Left ==
  InertFrmCg : Inport
  BdyFrmCg : Inport  Port=2
  HPbar : Inport  Port=3
  Hard Point Coordinate Transform External Displacement : autolibsharedcommon/Hard Point Coordinate Transform External Displacement  aMode=aMode
      settings: SourceProductName=Powertrain Blockset  SourceProductBaseCode=PW
  Selector1 : Selector  NumberOfDimensions=2  InputPortWidth=3  IndexOptions=Select all,Index vector (dialog)  Indices=[1],[3]  OutputSizes=1,1
  Inert : Outport
  Body : Outport  Port=2
  wires:
  InertFrmCg/1 -> Hard Point Coordinate Transform External Displacement/1
  Hard Point Coordinate Transform External Displacement/2 -> Body/1
  BdyFrmCg/1 -> Hard Point Coordinate Transform External Displacement/2
  Hard Point Coordinate Transform External Displacement/1 -> Inert/1
  HPbar/1 -> Selector1/1
  Selector1/1 -> Hard Point Coordinate Transform External Displacement/3

== system vehdynlibeom_TUM/Vehicle Body 6DOF/Signal Routing/Hard Point Coordinate Transform Rear Right ==
  InertFrmCg : Inport
  BdyFrmCg : Inport  Port=2
  HPbar : Inport  Port=3
  Hard Point Coordinate Transform External Displacement : autolibsharedcommon/Hard Point Coordinate Transform External Displacement  aMode=aMode
      settings: SourceProductName=Powertrain Blockset  SourceProductBaseCode=PW
  Selector1 : Selector  NumberOfDimensions=2  InputPortWidth=3  IndexOptions=Select all,Index vector (dialog)  Indices=[1],[4]  OutputSizes=1,1
  Inert : Outport
  Body : Outport  Port=2
  wires:
  Hard Point Coordinate Transform External Displacement/1 -> Inert/1
  BdyFrmCg/1 -> Hard Point Coordinate Transform External Displacement/2
  Hard Point Coordinate Transform External Displacement/2 -> Body/1
  InertFrmCg/1 -> Hard Point Coordinate Transform External Displacement/1
  HPbar/1 -> Selector1/1
  Selector1/1 -> Hard Point Coordinate Transform External Displacement/3

== system vehdynlibeom_TUM/Vehicle Body 6DOF/SignalCollection/phidot thetadot psidot ==
  phi theta psi : Inport
  p q r : Inport  Port=2
  Mux1 : Mux  Inputs=[3 3 3]
  Mux2 : Mux  Inputs=3
  phidot : Fcn  Expr=u[1]+(u[2]*u[4]+u[3]*u[7])*(u[5]/u[8])
  psidot : Fcn  Expr=(u[2]*u[4]+u[3]*u[7])/u[8]
  sincos : Trigonometry  Operator=sincos
  thetadot : Fcn  Expr=u[2]*u[7]-u[3]*u[4]
  phidot thetadot psidot : Outport  InitialOutput=0
  wires:
  Mux1/1 -> psidot/1, phidot/1, thetadot/1
  p q r/1 -> Mux1/1
  phi theta psi/1 -> sincos/1
  psidot/1 -> Mux2/3
  thetadot/1 -> Mux2/2
  phidot/1 -> Mux2/1
  Mux2/1 -> phidot thetadot psidot/1
  sincos/1 -> Mux1/2
  sincos/2 -> Mux1/3

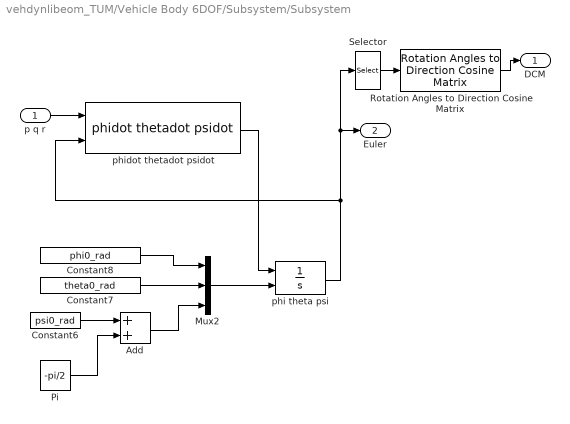
== system vehdynlibeom_TUM/Vehicle Body 6DOF/Subsystem/Subsystem ==
  "p q r " : Inport
  Add : Sum
  Constant6 : Constant  Value=psi0_rad
  Constant7 : Constant  Value=theta0_rad
  Constant8 : Constant  Value=phi0_rad
  Mux2 : Mux  Inputs=3
  Pi : Constant  Value=-pi/2  OutDataTypeStr=Inherit: Inherit via back propagation
  Rotation Angles to Direction Cosine Matrix : sharedtransform/Rotation Angles to Direction Cosine Matrix  rotationOrder=ZYX  aMode=aMode
      settings: SourceProductBaseCode=AE
  Selector : Selector  InputPortWidth=3  IndexOptions=Index vector (dialog)  Indices=[3 2 1]  OutputSizes=1
  phi theta psi : Integrator  InitialConditionSource=external  InitialCondition=[0,0,0]  WrapState=on
  phidot thetadot psidot : shared6dofsys/DCM & Euler Angles (Euler)/phidot thetadot psidot  SystemSampleTime=-1
      settings: SourceProductName=Aerospace Blockset  SourceProductBaseCode=AE
  DCM : Outport
  Euler : Outport  Port=2
  wires:
  phidot thetadot psidot/1 -> phi theta psi/1
  "p q r "/1 -> phidot thetadot psidot/1
  Selector/1 -> Rotation Angles to Direction Cosine Matrix/1
  phi theta psi/1 -> Selector/1, Euler/1, phidot thetadot psidot/2
  Rotation Angles to Direction Cosine Matrix/1 -> DCM/1
  Constant8/1 -> Mux2/1
  Constant7/1 -> Mux2/2
  Mux2/1 -> phi theta psi/2
  Pi/1 -> Add/2
  Constant6/1 -> Add/1
  Add/1 -> Mux2/3

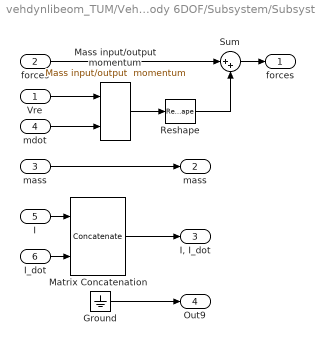
== system vehdynlibeom_TUM/Vehicle Body 6DOF/Subsystem/Subsystem1 ==
  Vre : Inport
  forces : Inport  Port=2
  "mass " : Inport  Port=3
  mdot : Inport  Port=4
  I : Inport  Port=5
  I_dot : Inport  Port=6
  Ground : Ground
  Mass input/output momentum : shared6dofsys/Mass & Inertia (custom)/Mass input//output  momentum  SystemSampleTime=-1
      settings: SourceProductName=Aerospace Blockset  SourceProductBaseCode=AE
  Matrix Concatenation : Concatenate  Mode=Multidimensional array
  Reshape : Reshape
  Sum : Sum  Inputs=|++  SaturateOnIntegerOverflow=on
  "forces " : Outport  PortDimensions=3
  mass : Outport  Port=2
  "I, I_dot " : Outport  Port=3
  Out9 : Outport  Port=4
  wires:
  Reshape/1 -> Sum/2
  Mass input/output momentum/1 -> Reshape/1
  I_dot/1 -> Matrix Concatenation/2
  Sum/1 -> "forces "/1
  forces/1 -> Sum/1
  "mass "/1 -> mass/1
  Vre/1 -> Mass input/output momentum/1
  I/1 -> Matrix Concatenation/1
  Matrix Concatenation/1 -> "I, I_dot "/1
  Ground/1 -> Out9/1
  mdot/1 -> Mass input/output momentum/2

== matlab function vehdynlibeom_TUM/Vehicle Body 6DOF/vehdyncginert ==
  data: m parameter size=1; Mbar output size=1; z1m parameter size=1; z2m parameter size=1; z3m parameter size=1; z4m parameter size=1; z5m parameter size=1; z6m parameter size=1; z7m parameter size=1; z1R parameter size=[1,3]; z2R parameter size=[1,3]; z3R parameter size=[1,3]; z4R parameter size=[1,3]; z5R parameter size=[1,3]; z6R parameter size=[1,3]; Iveh parameter size=[3,3]; z1I parameter size=[3,3]; z2I parameter size=[3,3]; z3I parameter size=[3,3]; z4I parameter size=[3,3]; z5I parameter size=[3,3]; z6I parameter size=[3,3]; z7I parameter size=[3,3]; Ibar output size=[3,3]; Rbar output; z7R parameter size=[1,3]; Xbar output; Wbar output; a parameter size=1; b parameter size=1; h parameter size=1; d parameter; HPbar output size=[3,4]; tw input size=2
function [Mbar,Ibar,Rbar,Xbar,Wbar,HPbar] = inert(m, z1m, z2m, z3m, z4m, z5m, z6m, z7m,z1R, z2R, z3R, z4R, z5R, z6R, Iveh, z1I, z2I, z3I, z4I, z5I, z6I, z7I, z7R, a, b, h, d, tw)%#codegen
coder.allowpcode('plain')

[Rbar,Mbar,Ibar,Xbar,Wbar,HPbar]= vehdyncginerthp(m, z1m, z2m, z3m, z4m, z5m, z6m, z7m,z1R, z2R, z3R, z4R, z5R, z6R, Iveh, z1I, z2I, z3I, z4I, z5I, z6I, z7I, z7R, a, b, h, tw, d);
end
